simulink model "OpenLoopWindTurbineModel_LinearVsNonlinear2014"  (R2017a)
settings: Solver=ode4  StartTime=0.0  StopTime=TIME_SIM  FixedStep=STEP_SIZE  MaxStep=0.001  RelTol=1e-6
values from neighbouring files (symbols this model uses):
  A = 13069.8108371    [OpenLoopWindTurbine_Parameters.mat]
  Bd = 6215000    [OpenLoopWindTurbine_Parameters.mat]
  beta_OP = 0.306891078961    [OpenLoopWindTurbine_OperatingPoint.mat]    (also in OpenLoopWindTurbine_Parameters.mat = 0.296705972839)
  CP0 = [0 0 0 0 0 0 0 0.0108523229163 0.0383908516897 0.0728169712581 0.106247295944 0.131224189854 ... (2500 elements, 50x50)]    [OpenLoopWindTurbine_Parameters.mat]
  Jg = 534.116    [OpenLoopWindTurbine_Parameters.mat]
  Jr = 59157000    [OpenLoopWindTurbine_Parameters.mat]
  Kd = 867637000    [OpenLoopWindTurbine_Parameters.mat]
  Lambda0 = [0.5 0.948979591837 1.39795918367 1.84693877551 2.29591836735 2.74489795918 3.19387755102 3.64285714286 4.09183673469 4.54081632653 4.98979591837 5.4387755102 ... (50 elements, 50x1)]    [OpenLoopWindTurbine_Parameters.mat]
  Ng = 97    [OpenLoopWindTurbine_Parameters.mat]
  Pitch0 = [-10 -9.18367346939 -8.36734693878 -7.55102040816 -6.73469387755 -5.91836734694 -5.10204081633 -4.28571428571 -3.4693877551 -2.65306122449 -1.83673469388 -1.02040816327 ... (50 elements, 50x1)]    [OpenLoopWindTurbine_Parameters.mat]
  R = 64.5    [OpenLoopWindTurbine_Parameters.mat]
  rho_air = 1.225    [OpenLoopWindTurbine_Parameters.mat]
  StepFinalValue_pitch = 0.296705972839    [OpenLoopWindTurbine_Parameters.mat]
  StepFinalValue_wind = 20    [OpenLoopWindTurbine_Parameters.mat]
  StepTime_pitch = 500    [OpenLoopWindTurbine_Parameters.mat]
  StepTime_wind = 500    [OpenLoopWindTurbine_Parameters.mat]
  Tg_OP = 40680.3126247    [OpenLoopWindTurbine_OperatingPoint.mat]    (also in OpenLoopWindTurbine_Parameters.mat)
  v_OP = 20    [OpenLoopWindTurbine_OperatingPoint.mat]    (also in OpenLoopWindTurbine_Parameters.mat)
  x0 = [1.26710910183 122.909582878 0.00454797377773]    [OpenLoopWindTurbine_OperatingPoint.mat]
undefined symbols (not defined in the file or in its folder): Aol, Bol, Bv, Col, Dol, u0, y0
settings Model: Creator=roga  LastModifiedBy=Roberto
settings DataIOCC: ExternalInput=[]  InitialState=[]  LimitDataPoints=on  LoadExternalInput=on  LoadInitialState=on  SaveFormat=Array
settings OptimizationCC: DefaultParameterBehavior=Inlined  BufferReuse=off  LifeSpan=inf
settings DebuggingCC: UnderspecifiedInitializationDetection=Classic  MergeDetectMultiDrivingBlocksExec=none  SolverPrmCheckMsg=warning  StateNameClashWarn=warning  InitInArrayFormatMsg=none  SFUnexpectedBacktrackingDiag=warning  SFNoUnconditionalDefaultTransitionDiag=warning  SFExecutionAtInitializationDiag=none
settings HardwareCC: ProdBitPerPointer=32  ProdBitPerSizeT=32  ProdBitPerPtrDiffT=32  ProdLargestAtomicFloat=None  ProdIntDivRoundTo=Undefined  ProdEndianess=Unspecified  ProdWordSize=32  ProdHWDeviceType=32-bit Generic
settings ModelReferenceCC: PropagateSignalLabelsOutOfModel=off
settings GRTTargetCC: TargetLangStandard=C89/C90 (ANSI)  GeneratePreprocessorConditionals=Disable all
settings ConfigComp: CovMetricSettings=dw  CovHtmlReporting=on  CovSaveCumulativeToWorkspaceVar=on  CovSaveSingleToWorkspaceVar=on  CovExternalEMLEnable=off  CovSFcnEnable=off

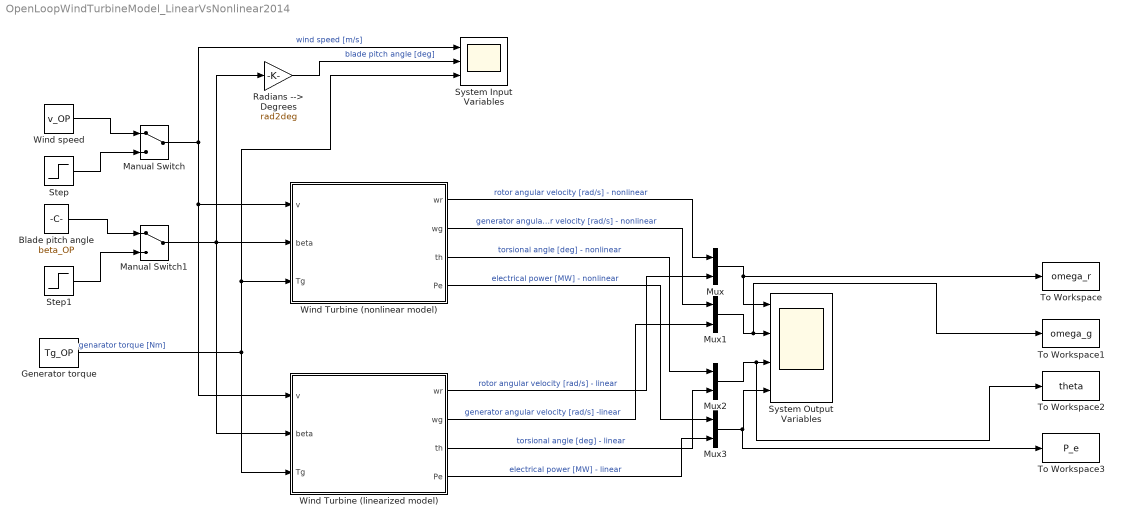
== system OpenLoopWindTurbineModel_LinearVsNonlinear2014 ==
  Blade pitch angle : Constant  Value=beta_OP
      mask Display: port_label('output',1,'\beta_{OP}','Interpreter','tex')
  Generator torque : Constant  Value=Tg_OP
      mask Display: port_label('output',1,'T_{g,OP}','Interpreter','tex')
  Manual Switch : ManualSwitch
  Manual Switch1 : ManualSwitch
  Mux{,1..3} (4 alike) : Mux  Inputs=2
  Radians --> Degrees : Gain  Gain=rad2deg
  Step : Step  Time=StepTime_wind  Before=v_OP  After=StepFinalValue_wind  SampleTime=0
  Step1 : Step  Time=StepTime_pitch  Before=beta_OP  After=StepFinalValue_pitch  SampleTime=0
  System Input Variables : Scope  NumInputPorts=3
  System Output Variables : Scope  NumInputPorts=4
  To Workspace : ToWorkspace  VariableName=omega_r  SaveFormat=Structure With Time  SampleTime=-1
  To Workspace1 : ToWorkspace  VariableName=omega_g  SaveFormat=Structure With Time  SampleTime=-1
  To Workspace2 : ToWorkspace  VariableName=theta  SaveFormat=Structure With Time  SampleTime=-1
  To Workspace3 : ToWorkspace  VariableName=P_e  SaveFormat=Structure With Time  SampleTime=-1
  Wind Turbine (linearized model) : Subsystem
      mask Display:
      | image('wind_turbine.jpg')
      | port_label('input',1,'v')
      | port_label('input',2,'\beta','Interpreter','tex')
      | port_label('input',3,'T_g','Interpreter','tex')
      | port_label('output',1,'\omega_r','Interpreter','tex')
      | port_label('output',2,'\omega_g','Interpreter','tex')
      | port_label('output',3,'\theta','Interpreter','tex')
      | port_label('output',4,'P_e','Interpreter','tex')
  Wind Turbine (nonlinear model) : Subsystem
      mask Display:
      | image('wind_turbine.jpg')
      | port_label('input',1,'v')
      | port_label('input',2,'\beta','Interpreter','tex')
      | port_label('input',3,'T_g','Interpreter','tex')
      | port_label('output',1,'\omega_r','Interpreter','tex')
      | port_label('output',2,'\omega_g','Interpreter','tex')
      | port_label('output',3,'\theta','Interpreter','tex')
      | port_label('output',4,'P_e','Interpreter','tex')
  Wind speed : Constant  Value=v_OP
      mask Display: port_label('output',1,'v_{OP}','Interpreter','tex')
  wires:
  Mux/1 -> To Workspace/1, System Output Variables/1
  Mux1/1 -> To Workspace1/1, System Output Variables/2
  Mux2/1 -> To Workspace2/1, System Output Variables/3
  Mux3/1 -> To Workspace3/1, System Output Variables/4
  Wind Turbine (nonlinear model)/1(wr) -> Mux/1  "rotor angular velocity [rad/s] - nonlinear"
  Wind Turbine (linearized model)/1(wr) -> Mux/2  "rotor angular velocity [rad/s] - linear"
  Wind Turbine (nonlinear model)/2(wg) -> Mux1/1  "generator angular velocity [rad/s] - nonlinear"
  Wind Turbine (linearized model)/2(wg) -> Mux1/2  "generator angular velocity [rad/s] -linear"
  Wind Turbine (nonlinear model)/3(th) -> Mux2/1  "torsional angle [deg] - nonlinear"
  Wind Turbine (linearized model)/3(th) -> Mux2/2  "torsional angle [deg] - linear"
  Wind Turbine (nonlinear model)/4(Pe) -> Mux3/1  "electrical power [MW] - nonlinear"
  Wind Turbine (linearized model)/4(Pe) -> Mux3/2  "electrical power [MW] - linear"
  Radians --> Degrees/1 -> System Input Variables/2  "blade pitch angle [deg]"
  Wind speed/1 -> Manual Switch/1
  Manual Switch/1 -> Wind Turbine (linearized model)/1(v), Wind Turbine (nonlinear model)/1(v), System Input Variables/1  "wind speed [m/s]"
  Manual Switch1/1 -> Wind Turbine (linearized model)/2(beta), Radians --> Degrees/1, Wind Turbine (nonlinear model)/2(beta)
  Blade pitch angle/1 -> Manual Switch1/1
  Step/1 -> Manual Switch/2
  Step1/1 -> Manual Switch1/2
  Generator torque/1 -> Wind Turbine (linearized model)/3(Tg), System Input Variables/3, Wind Turbine (nonlinear model)/3(Tg)  "genarator torque [Nm]"

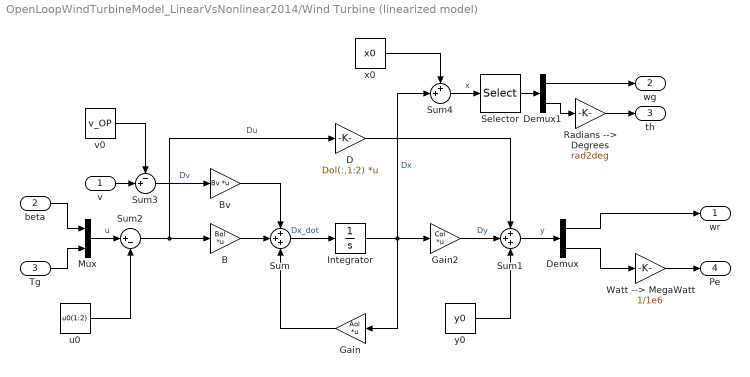
== system OpenLoopWindTurbineModel_LinearVsNonlinear2014/Wind Turbine (linearized model) ==
  v : Inport
  beta : Inport  Port=2
  Tg : Inport  Port=3
  B : Gain  Gain=Bol  Multiplication=Matrix(K*u) (u vector)
  Bv : Gain  Gain=Bv  Multiplication=Matrix(K*u) (u vector)
  D : Gain  Gain=Dol(:,1:2)  Multiplication=Matrix(K*u) (u vector)
  Demux : Demux  Outputs=2
  Demux1 : Demux  Outputs=2
  Gain : Gain  Gain=Aol  Multiplication=Matrix(K*u) (u vector)
  Gain2 : Gain  Gain=Col  Multiplication=Matrix(K*u) (u vector)
  Integrator : Integrator  InitialCondition=zeros(3,1)
  Mux : Mux  Inputs=2
  Radians --> Degrees : Gain  Gain=rad2deg
  Selector : Selector  InputPortWidth=3  IndexOptions=Index vector (dialog)  Indices=[2 3]  OutputSizes=1
  Sum : Sum  Inputs=+++
  Sum1 : Sum  Inputs=+++
  Sum2 : Sum  Inputs=|+-
  Sum3 : Sum  Inputs=-+|
  Sum4 : Sum  Inputs=++|
  Watt --> MegaWatt : Gain  Gain=1/1e6
  u0 : Constant  Value=u0(1:2)
  v0 : Constant  Value=v_OP
  x0 : Constant  Value=x0
  y0 : Constant  Value=y0
  wr : Outport
  wg : Outport  Port=2
  th : Outport  Port=3
  Pe : Outport  Port=4
  wires:
  Integrator/1 -> Sum4/2, Gain/1, Gain2/1  "Dx"
  u0/1 -> Sum2/2
  Sum/1 -> Integrator/1  "Dx_dot"
  Gain/1 -> Sum/3
  Gain2/1 -> Sum1/2  "Dy"
  Bv/1 -> Sum/1
  D/1 -> Sum1/1
  B/1 -> Sum/2
  Sum1/1 -> Demux/1  "y"
  beta/1 -> Mux/1
  Tg/1 -> Mux/2
  y0/1 -> Sum1/3
  Sum2/1 -> D/1, B/1  "Du"
  Mux/1 -> Sum2/1  "u"
  Sum3/1 -> Bv/1  "Dv"
  v/1 -> Sum3/2
  v0/1 -> Sum3/1
  Selector/1 -> Demux1/1
  Sum4/1 -> Selector/1  "x"
  x0/1 -> Sum4/1
  Demux1/1 -> wg/1
  Demux1/2 -> Radians --> Degrees/1
  Demux/1 -> wr/1
  Demux/2 -> Watt --> MegaWatt/1
  Radians --> Degrees/1 -> th/1
  Watt --> MegaWatt/1 -> Pe/1

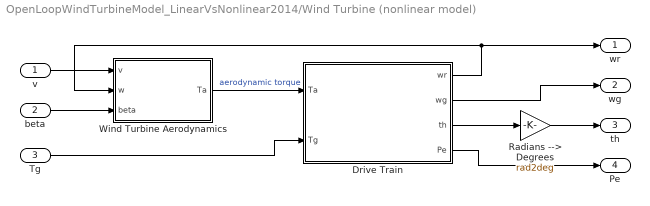
== system OpenLoopWindTurbineModel_LinearVsNonlinear2014/Wind Turbine (nonlinear model) ==
  v : Inport
  beta : Inport  Port=2
  Tg : Inport  Port=3
  Drive Train : Subsystem
      mask Display:
      | image('wind_turbine_nacelle.jpg')
      | port_label('input',1,'T_a','Interpreter','tex')
      | port_label('input',2,'T_g','Interpreter','tex')
      | port_label('output',1,'\omega_r','Interpreter','tex')
      | port_label('output',2,'\omega_g','Interpreter','tex')
      | port_label('output',3,'\theta','Interpreter','tex')
      | port_label('output',4,'P_e','Interpreter','tex')
  Radians --> Degrees : Gain  Gain=rad2deg
  Wind Turbine Aerodynamics : Subsystem
      mask Display:
      | image('PowerCoefficient.jpg')
      | port_label('input',1,'v')
      | port_label('input',2,'\omega_r','Interpreter','tex')
      | port_label('input',3,'\beta','Interpreter','tex')
      | port_label('output',1,'T_a','Interpreter','tex')
  wr : Outport
  wg : Outport  Port=2
  th : Outport  Port=3
  Pe : Outport  Port=4
  wires:
  Drive Train/1(wr) -> wr/1, Wind Turbine Aerodynamics/2(w)
  Tg/1 -> Drive Train/2(Tg)
  Drive Train/2(wg) -> wg/1
  Drive Train/3(th) -> Radians --> Degrees/1
  Drive Train/4(Pe) -> Pe/1
  beta/1 -> Wind Turbine Aerodynamics/3(beta)
  Wind Turbine Aerodynamics/1(Ta) -> Drive Train/1(Ta)  "aerodynamic torque"
  v/1 -> Wind Turbine Aerodynamics/1(v)
  Radians --> Degrees/1 -> th/1

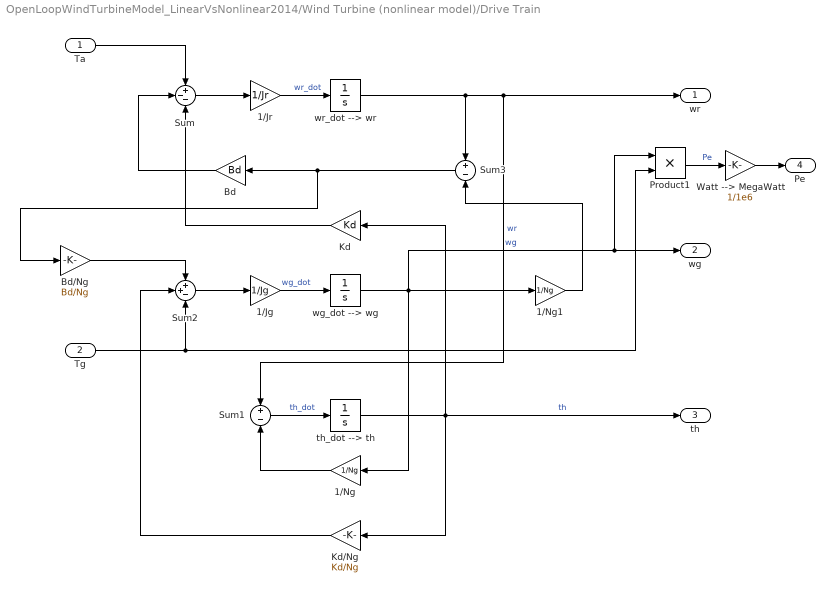
== system OpenLoopWindTurbineModel_LinearVsNonlinear2014/Wind Turbine (nonlinear model)/Drive Train ==
  Ta : Inport
  Tg : Inport  Port=2
  1/Jg : Gain  Gain=1/Jg
  1/Jr : Gain  Gain=1/Jr
  1/Ng : Gain  Gain=1/Ng
  1/Ng1 : Gain  Gain=1/Ng
  Bd : Gain  Gain=Bd
  Bd/Ng : Gain  Gain=Bd/Ng
  Kd : Gain  Gain=Kd
  Kd/Ng : Gain  Gain=Kd/Ng
  Product1 : Product
  Sum : Sum  Inputs=+--
  Sum1 : Sum  Inputs=+-
  Sum2 : Sum  Inputs=++-
  Sum3 : Sum  Inputs=+-
  Watt --> MegaWatt : Gain  Gain=1/1e6
  th_dot --> th : Integrator  Priority=3  InitialCondition=x0(3)  LowerSaturationLimit=0
  wg_dot --> wg : Integrator  Priority=2  InitialCondition=x0(2)  LowerSaturationLimit=0
  wr_dot --> wr : Integrator  Priority=1  InitialCondition=x0(1)  LowerSaturationLimit=0
  wr : Outport
  wg : Outport  Port=2
  th : Outport  Port=3
  Pe : Outport  Port=4
  wires:
  wg_dot --> wg/1 -> Product1/1, wg/1, 1/Ng1/1, 1/Ng/1  "wg"
  wr_dot --> wr/1 -> Sum3/1, wr/1, Sum1/1  "wr"
  1/Ng/1 -> Sum1/2
  Sum1/1 -> th_dot --> th/1  "th_dot"
  Sum2/1 -> 1/Jg/1
  1/Ng1/1 -> Sum3/2
  Sum/1 -> 1/Jr/1
  1/Jr/1 -> wr_dot --> wr/1  "wr_dot"
  th_dot --> th/1 -> th/1, Kd/Ng/1, Kd/1  "th"
  1/Jg/1 -> wg_dot --> wg/1  "wg_dot"
  Sum3/1 -> Bd/Ng/1, Bd/1
  Bd/1 -> Sum/2
  Kd/1 -> Sum/3
  Bd/Ng/1 -> Sum2/1
  Kd/Ng/1 -> Sum2/2
  Ta/1 -> Sum/1
  Tg/1 -> Product1/2, Sum2/3
  Product1/1 -> Watt --> MegaWatt/1  "Pe"
  Watt --> MegaWatt/1 -> Pe/1

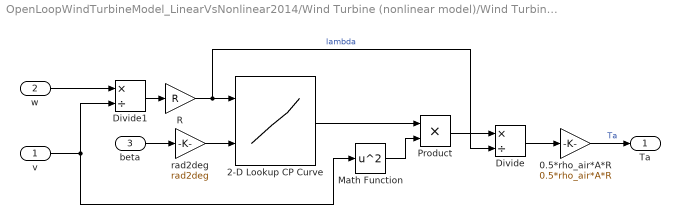
== system OpenLoopWindTurbineModel_LinearVsNonlinear2014/Wind Turbine (nonlinear model)/Wind Turbine Aerodynamics ==
  v : Inport
  w : Inport  Port=2
  beta : Inport  Port=3
  0.5*rho_air*A*R : Gain  Gain=0.5*rho_air*A*R
  2-D Lookup CP Curve : Lookup_n-D  BreakpointsForDimension1=Lambda0  BreakpointsForDimension2=Pitch0  BreakpointsForDimension3=CP0'  Table=CP0  DiagnosticForOutOfRangeInput=Warning  RndMeth=Simplest  InputSameDT=on
  Divide : Product  Inputs=*/
  Divide1 : Product  Inputs=*/
  Math Function : Math  Operator=square  SaturateOnIntegerOverflow=on
  Product : Product
  R : Gain  Gain=R
  rad2deg : Gain  Gain=rad2deg
  Ta : Outport
  wires:
  0.5*rho_air*A*R/1 -> Ta/1  "Ta"
  beta/1 -> rad2deg/1
  w/1 -> Divide1/1
  Divide/1 -> 0.5*rho_air*A*R/1
  Product/1 -> Divide/1
  Math Function/1 -> Product/2
  2-D Lookup CP Curve/1 -> Product/1
  v/1 -> Divide1/2, Math Function/1
  Divide1/1 -> R/1
  R/1 -> Divide/2, 2-D Lookup CP Curve/1  "lambda"
  rad2deg/1 -> 2-D Lookup CP Curve/2
